simulink model "MLI"  (R2016a)
settings: Solver=VariableStepAuto  StartTime=0.0  StopTime=10  RelTol=1e-3
libraries: powerlib x26, powerlib_meascontrol x5, simulink x1
settings Model: Creator=Alin anto  LastModifiedBy=Alin anto

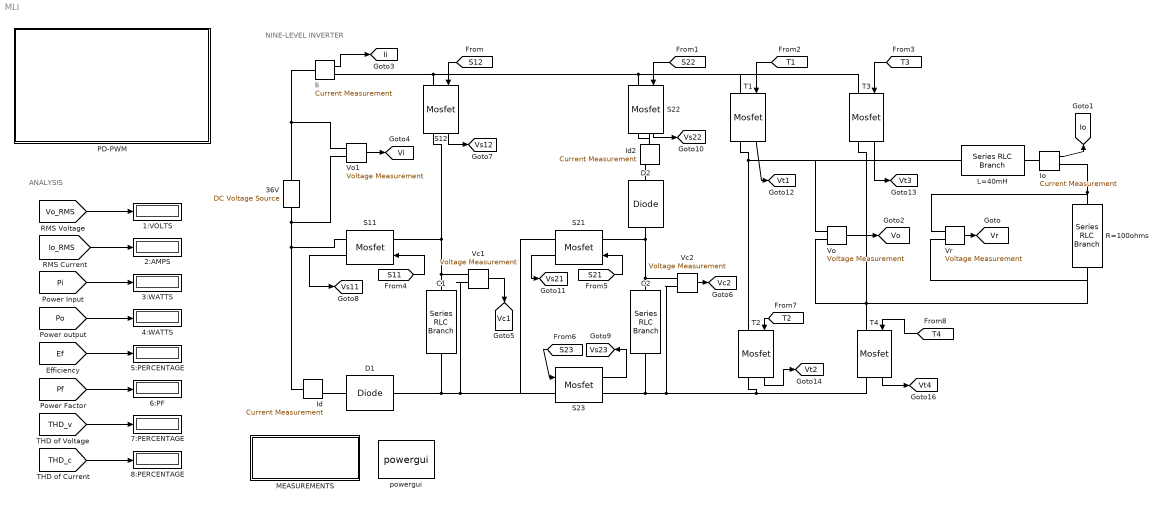
== system MLI ==
  note: ANALYSIS
  note: NINE-LEVEL INVERTER
  1:VOLTS : Display
  2:AMPS : Display
  36V : powerlib/Electrical Sources/DC Voltage Source  Amplitude=36  Measurements=None
  3:WATTS : Display
  4:WATTS : Display
  5:PERCENTAGE : Display
  6:PF : Display
  7:PERCENTAGE : Display
  8:PERCENTAGE : Display
  C1 : powerlib/Elements/Series RLC Branch  LConnTagsString=__new0  RConnTagsString=__new0  BranchType=C  Resistance=1  Inductance=1e-3  SetiL0=off  InitialCurrent=0  Capacitance=0.0024  Setx0=off  InitialVoltage=0  Measurements=None
  C2 : powerlib/Elements/Series RLC Branch  LConnTagsString=__new0  RConnTagsString=__new0  BranchType=C  Resistance=1  Inductance=1e-3  SetiL0=off  InitialCurrent=0  Capacitance=0.0036  Setx0=off  InitialVoltage=0  Measurements=None
  D1 : powerlib/Power Electronics/Diode  Ron=0.001  Lon=0  Vf=0.8  IC=0  UseSnubber=off  Rs=500  Cs=250e-9  Measurements=off
  D2 : powerlib/Power Electronics/Diode  Ron=0.001  Lon=0  Vf=0.8  IC=0  UseSnubber=off  Rs=500  Cs=250e-9  Measurements=off
  Id : powerlib/Measurements/Current Measurement  PhasorSimulation=off  OutputType=Complex  PSBequivalent=0
  Id2 : powerlib/Measurements/Current Measurement  PhasorSimulation=off  OutputType=Complex  PSBequivalent=0
  Ii : powerlib/Measurements/Current Measurement  PhasorSimulation=off  OutputType=Complex  PSBequivalent=0
  Io : powerlib/Measurements/Current Measurement  PhasorSimulation=off  OutputType=Complex  PSBequivalent=0
  L=40mH : powerlib/Elements/Series RLC Branch  LConnTagsString=__new0  RConnTagsString=__new0  BranchType=L  Resistance=1  Inductance=0.040  SetiL0=off  InitialCurrent=0  Capacitance=1e-6  Setx0=off  InitialVoltage=0  Measurements=None
  MEASUREMENTS : Subsystem
  PD-PWM : Subsystem
  R=100ohms : powerlib/Elements/Series RLC Branch  LConnTagsString=__new0  RConnTagsString=__new0  BranchType=R  Resistance=100  Inductance=1e-3  SetiL0=off  InitialCurrent=0  Capacitance=1e-6  Setx0=off  InitialVoltage=0  Measurements=None
  S{11..12,21..23} (5 alike) : powerlib/Power Electronics/Mosfet  Ron=0.1  Lon=0  Rd=0.01  Vfd=0.7  IC=0  Rs=1e5  Cs=inf  Measurements=on
  T{1..4} (4 alike) : powerlib/Power Electronics/Mosfet  Ron=0.1  Lon=0  Rd=0.01  Vfd=0.7  IC=0  Rs=1e5  Cs=inf  Measurements=on
  Vc1 : powerlib/Measurements/Voltage Measurement  PhasorSimulation=off  OutputType=Complex  PSBequivalent=0
  Vc2 : powerlib/Measurements/Voltage Measurement  PhasorSimulation=off  OutputType=Complex  PSBequivalent=0
  Vo : powerlib/Measurements/Voltage Measurement  PhasorSimulation=off  OutputType=Complex  PSBequivalent=0
  Vo1 : powerlib/Measurements/Voltage Measurement  PhasorSimulation=off  OutputType=Complex  PSBequivalent=0
  Vr : powerlib/Measurements/Voltage Measurement  PhasorSimulation=off  OutputType=Complex  PSBequivalent=0
  powergui : powerlib/powergui  Priority=1  SimulationMode=Discrete  SolverType=Tustin/Backward Euler (TBE)  SampleTime=1e-6  frequency=60  SPID=off  DisableSnubberDevices=off  DisableRonSwitches=off  DisableVfSwitches=off  SwTol=0  DisplayEquations=off  Interpol=off  ExternalGateDelay=off  methode=off  Ts=10  FunctionMessages=off  echomessages=off  HookPort=off  EnableUseOfTLC=off  x0status=blocks  frequencyindice=0  Pbase=100e6  ErrMax=1e-4  Iterations=50  UnitsV=kV  UnitsW=MW  buscounter=0  RestoreLinks=warning  ResistiveCurrentMeasurement=off  Frange=[0:2:500]  Ylog=off  Xlog=on  ShowGrid=off  save=off  variable=ZData  structure=FFT  ZoomFFT=on  StartTime=0.3  cycles=5  DisplayStyle=1  fundamental=50  FreqAxis=off  MaxFrequency=10000  frequencyindicesteady=1  RmsSteady=1  display=off
  tag scope: Ii=global, Io=global, Vc1=global, Vc2=global, Vi=global, Vo=global, Vr=global, Vs11=global, Vs12=global, Vs21=global, Vs22=global, Vs23=global, Vt1=global, Vt2=global, Vt3=global, Vt4=global
  wires:
  [T2] -> T2/1
  [S22] -> S22/1
  [S21] -> S21/1
  [T4] -> T4/1
  [S12] -> S12/1
  [S23] -> S23/1
  [T1] -> T1/1
  [S11] -> S11/1
  [T3] -> T3/1
  Io/1 -> [Io]
  Vo/1 -> [Vo]
  Vr/1 -> [Vr]
  Ii/1 -> [Ii]
  Vo1/1 -> [Vi]
  [Pi] -> 3:WATTS/1
  [THD_v] -> 7:PERCENTAGE/1
  [Pf] -> 6:PF/1
  [Ef] -> 5:PERCENTAGE/1
  [Po] -> 4:WATTS/1
  [THD_c] -> 8:PERCENTAGE/1
  [Io_RMS] -> 2:AMPS/1
  [Vo_RMS] -> 1:VOLTS/1
  Vc2/1 -> [Vc2]
  Vc1/1 -> [Vc1]
  S12/1 -> [Vs12]
  S11/1 -> [Vs11]
  S23/1 -> [Vs23]
  S22/1 -> [Vs22]
  S21/1 -> [Vs21]
  T4/1 -> [Vt4]
  T2/1 -> [Vt2]
  T1/1 -> [Vt1]
  T3/1 -> [Vt3]
  connections:
  S12/LConn1 -- Ii/RConn1 -- T3/LConn1 -- T1/LConn1 -- S22/LConn1
  L=40mH/RConn1 -- Io/LConn1
  T1/RConn1 -- Vo/LConn1 -- L=40mH/LConn1 -- T2/LConn1
  S23/RConn1 -- C2/RConn1 -- Vc2/LConn2 -- T2/RConn1 -- T4/RConn1
  36V/LConn1 -- Vo1/LConn2 -- Id/LConn1 -- S11/RConn1
  D1/LConn1 -- S21/RConn1 -- S23/LConn1 -- Vc1/LConn2 -- C1/RConn1
  C1/LConn1 -- S11/LConn1 -- S12/RConn1 -- Vc1/LConn1
  C2/LConn1 -- Vc2/LConn1 -- D2/RConn1 -- S21/LConn1
  Io/RConn1 -- Vr/LConn1 -- R=100ohms/LConn1
  T3/RConn1 -- R=100ohms/RConn1 -- Vr/LConn2 -- Vo/LConn2 -- T4/LConn1
  36V/RConn1 -- Vo1/LConn1 -- Ii/LConn1
  Id/RConn1 -- D1/RConn1
  Id2/RConn1 -- D2/LConn1
  Id2/LConn1 -- S22/RConn1

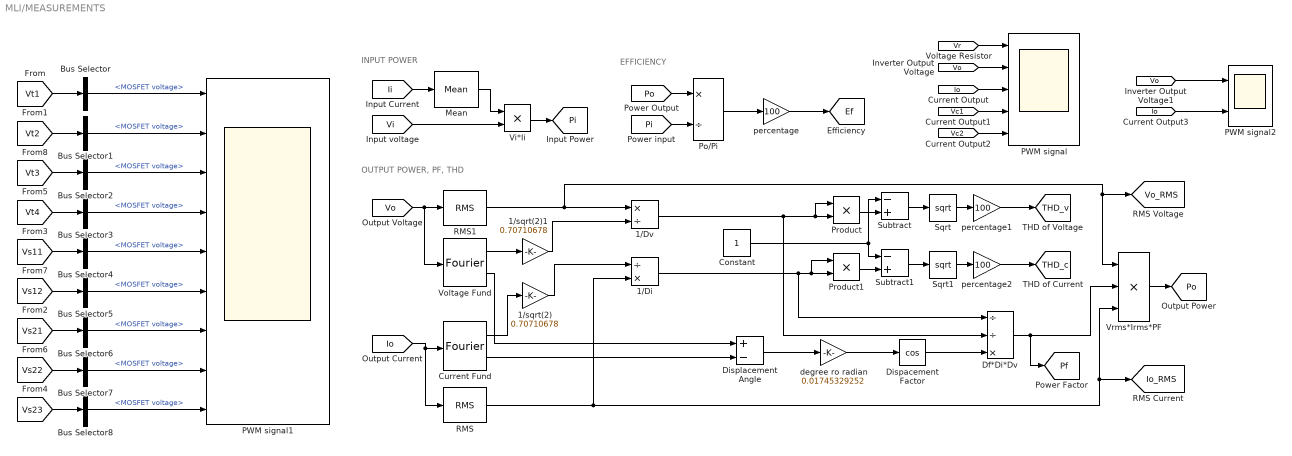
== system MLI/MEASUREMENTS ==
  note: OUTPUT POWER, PF, THD
  note: EFFICIENCY
  note: INPUT POWER
  1/Di : Product  Inputs=/*
  1/Dv : Product  Inputs=*/
  1/sqrt(2) : Gain  Gain=0.70710678
  1/sqrt(2)1 : Gain  Gain=0.70710678
  Bus Selector{,1..8} (9 alike) : BusSelector  OutputSignals=MOSFET voltage
  Constant : Constant
  Current Fund : powerlib_meascontrol/Measurements/Fourier  Freq=50  n=1  InInit=[120, 0]  Ts=0
  Df*Di*Dv : Product  Inputs=//*
  Dispacement Factor : Trigonometry  Operator=cos
  Displacement Angle : Sum  Inputs=+-
  Mean : powerlib_meascontrol/Measurements/Mean  Freq=50  Vinit=1  Ts=0
  PWM signal : Scope  NumInputPorts=5
  PWM signal1 : Scope  NumInputPorts=9
  PWM signal2 : Scope  NumInputPorts=2
  Po/Pi : Product  Inputs=*/
  Product : Product
  Product1 : Product
  RMS : powerlib_meascontrol/Measurements/RMS  TrueRMS=on  Freq=50  RMSInit=120  Ts=0
  RMS1 : powerlib_meascontrol/Measurements/RMS  TrueRMS=on  Freq=50  RMSInit=120  Ts=0
  Sqrt : Sqrt  SaturateOnIntegerOverflow=on
  Sqrt1 : Sqrt  SaturateOnIntegerOverflow=on
  Subtract : Sum  Inputs=-+
  Subtract1 : Sum  Inputs=-+
  Vi*Ii : Product
  Voltage Fund : powerlib_meascontrol/Measurements/Fourier  Freq=50  n=1  InInit=[120, 0]  Ts=0
  Vrms*Irms*PF : Product  Inputs=3
  degree ro radian : Gain  Gain=0.01745329252
  percentage : Gain  Gain=100
  percentage1 : Gain  Gain=100
  percentage2 : Gain  Gain=100
  tag scope: Ef=global, Io_RMS=global, Pf=global, Pi=global, Po=global, THD_c=global, THD_v=global, Vo_RMS=global
  wires:
  [Ii] -> Mean/1
  Mean/1 -> Vi*Ii/1
  [Vi] -> Vi*Ii/2
  Vi*Ii/1 -> [Pi]
  [Io] -> RMS/1, Current Fund/1
  Current Fund/1 -> 1/sqrt(2)/1
  RMS/1 -> [Io_RMS], Vrms*Irms*PF/3, 1/Di/2
  [Vo] -> Voltage Fund/1, RMS1/1
  Voltage Fund/1 -> 1/sqrt(2)1/1
  RMS1/1 -> [Vo_RMS], Vrms*Irms*PF/1, 1/Dv/1
  Voltage Fund/2 -> Displacement Angle/1
  Current Fund/2 -> Displacement Angle/2
  Displacement Angle/1 -> degree ro radian/1
  degree ro radian/1 -> Dispacement Factor/1
  1/Dv/1 -> Product/2, Product/1, Df*Di*Dv/2
  1/Di/1 -> Product1/1, Product1/2, Df*Di*Dv/1
  Df*Di*Dv/1 -> [Pf], Vrms*Irms*PF/2
  1/sqrt(2)1/1 -> 1/Dv/2
  Vrms*Irms*PF/1 -> [Po]
  Product/1 -> Subtract/2
  Constant/1 -> Subtract/1, Subtract1/1
  Subtract/1 -> Sqrt/1
  Subtract1/1 -> Sqrt1/1
  [Po] -> Po/Pi/1
  [Pi] -> Po/Pi/2
  Po/Pi/1 -> percentage/1
  percentage/1 -> [Ef]
  Sqrt/1 -> percentage1/1
  percentage1/1 -> [THD_v]
  Sqrt1/1 -> percentage2/1
  percentage2/1 -> [THD_c]
  [Vr] -> PWM signal/1
  [Vo] -> PWM signal/2
  [Io] -> PWM signal/3
  1/sqrt(2)/1 -> 1/Di/1
  Product1/1 -> Subtract1/2
  Dispacement Factor/1 -> Df*Di*Dv/3
  [Vc1] -> PWM signal/4
  [Vc2] -> PWM signal/5
  [Vt1] -> Bus Selector/1
  [Vt2] -> Bus Selector1/1
  [Vt3] -> Bus Selector2/1
  [Vt4] -> Bus Selector3/1
  [Vs11] -> Bus Selector4/1
  [Vs12] -> Bus Selector5/1
  [Vs21] -> Bus Selector6/1
  [Vs22] -> Bus Selector7/1
  [Vs23] -> Bus Selector8/1
  Bus Selector/1 -> PWM signal1/1  "<MOSFET voltage>"
  Bus Selector1/1 -> PWM signal1/2  "<MOSFET voltage>"
  Bus Selector2/1 -> PWM signal1/3  "<MOSFET voltage>"
  Bus Selector3/1 -> PWM signal1/4  "<MOSFET voltage>"
  Bus Selector4/1 -> PWM signal1/5  "<MOSFET voltage>"
  Bus Selector5/1 -> PWM signal1/6  "<MOSFET voltage>"
  Bus Selector6/1 -> PWM signal1/7  "<MOSFET voltage>"
  Bus Selector7/1 -> PWM signal1/8  "<MOSFET voltage>"
  Bus Selector8/1 -> PWM signal1/9  "<MOSFET voltage>"
  [Vo] -> PWM signal2/1
  [Io] -> PWM signal2/2

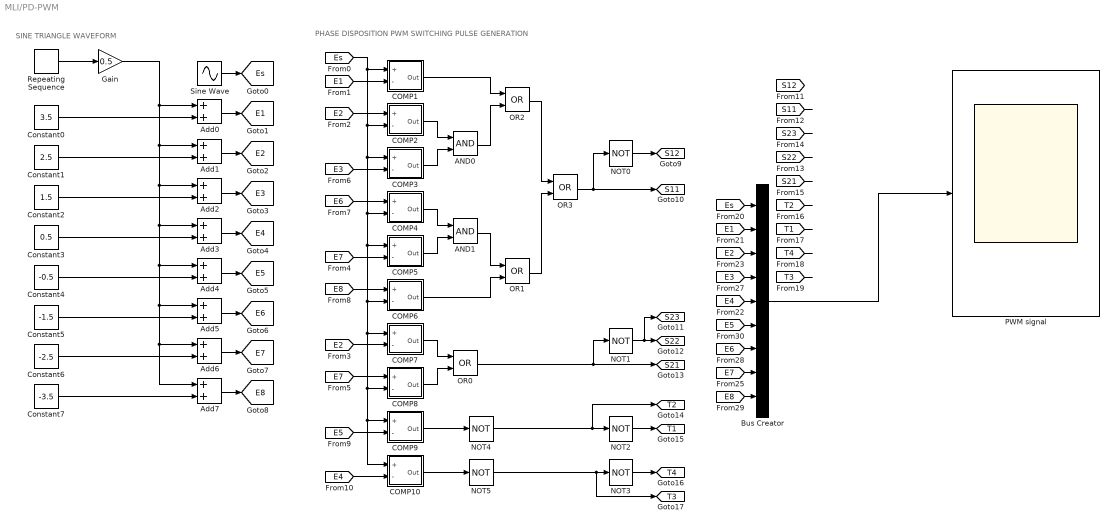
== system MLI/PD-PWM ==
  note: PHASE DISPOSITION PWM SWITCHING PULSE GENERATION
  note: SINE TRIANGLE WAVEFORM
  AND0 : Logic  AllPortsSameDT=off  OutDataTypeStr=boolean
  AND1 : Logic  AllPortsSameDT=off  OutDataTypeStr=boolean
  Add{0..7} (8 alike) : Sum
  Bus Creator : BusCreator  Inputs=9
  COMP1 : Subsystem
  COMP10 : Subsystem
  COMP2 : Subsystem
  COMP3 : Subsystem
  COMP4 : Subsystem
  COMP5 : Subsystem
  COMP6 : Subsystem
  COMP7 : Subsystem
  COMP8 : Subsystem
  COMP9 : Subsystem
  Constant0 : Constant  Value=3.5
  Constant1 : Constant  Value=2.5
  Constant2 : Constant  Value=1.5
  Constant3 : Constant  Value=0.5
  Constant4 : Constant  Value=-0.5
  Constant5 : Constant  Value=-1.5
  Constant6 : Constant  Value=-2.5
  Constant7 : Constant  Value=-3.5
  Gain : Gain  Gain=0.5
  NOT{0..5} (6 alike) : Logic  Operator=NOT  AllPortsSameDT=off  OutDataTypeStr=boolean
  OR{0..3} (4 alike) : Logic  Operator=OR  AllPortsSameDT=off  OutDataTypeStr=boolean
  PWM signal : Scope
  Repeating Sequence : simulink/Sources/Repeating Sequence  rep_seq_t=[0 5e-5 15e-5 20e-5]  rep_seq_y=[0 1 -1 0]
  Sine Wave : Sin  Amplitude=4  Frequency=2*pi*50  SampleTime=0
  tag scope: E1=global, E2=global, E3=global, E4=global, E5=global, E6=global, E7=global, E8=global, Es=global, S11=global, S12=global, S21=global, S22=global, S23=global, T1=global, T2=global, T3=global, T4=global
  wires:
  COMP1/1(Out) -> OR2/1
  OR0/1 -> [S21], NOT1/1
  OR3/1 -> [S11], NOT0/1
  OR2/1 -> OR3/1
  OR1/1 -> OR3/2
  NOT1/1 -> [S22], [S23]
  NOT0/1 -> [S12]
  COMP4/1(Out) -> AND1/1
  COMP7/1(Out) -> OR0/1
  COMP2/1(Out) -> AND0/1
  COMP6/1(Out) -> OR1/2
  AND0/1 -> OR2/2
  COMP3/1(Out) -> AND0/2
  COMP5/1(Out) -> AND1/2
  AND1/1 -> OR1/1
  COMP8/1(Out) -> OR0/2
  [Es] -> COMP4/2(-), COMP6/2(-), COMP7/1(+), COMP8/2(-), COMP9/1(+), COMP10/1(+), COMP5/1(+), COMP3/1(+), COMP2/2(-), COMP1/1(+)
  [E1] -> COMP1/2(-)
  [E2] -> COMP2/1(+)
  [E3] -> COMP3/2(-)
  [E6] -> COMP4/1(+)
  [E7] -> COMP5/2(-)
  [E8] -> COMP6/1(+)
  [E5] -> COMP9/2(-)
  [E4] -> COMP10/2(-)
  COMP9/1(Out) -> NOT4/1
  NOT4/1 -> [T2], NOT2/1
  NOT2/1 -> [T1]
  COMP10/1(Out) -> NOT5/1
  NOT5/1 -> [T3], NOT3/1
  NOT3/1 -> [T4]
  Constant2/1 -> Add2/2
  Constant3/1 -> Add3/2
  Constant0/1 -> Add0/2
  Constant1/1 -> Add1/2
  Repeating Sequence/1 -> Gain/1
  Gain/1 -> Add7/1, Add6/1, Add5/1, Add4/1, Add3/1, Add2/1, Add1/1, Add0/1
  Constant4/1 -> Add4/2
  Constant6/1 -> Add6/2
  Constant7/1 -> Add7/2
  Constant5/1 -> Add5/2
  Sine Wave/1 -> [Es]
  Add0/1 -> [E1]
  Add1/1 -> [E2]
  Add2/1 -> [E3]
  Add7/1 -> [E8]
  Add6/1 -> [E7]
  Add5/1 -> [E6]
  Add4/1 -> [E5]
  Add3/1 -> [E4]
  [E2] -> COMP7/2(-)
  [E7] -> COMP8/1(+)
  [S23] -> ?
  [S22] -> ?
  [S21] -> ?
  [T2] -> ?
  [T1] -> ?
  [T4] -> ?
  [T3] -> ?
  [S11] -> ?
  [Es] -> Bus Creator/1
  [E1] -> Bus Creator/2
  [E2] -> Bus Creator/3
  [E3] -> Bus Creator/4
  [E4] -> Bus Creator/5
  [E5] -> Bus Creator/6
  [E6] -> Bus Creator/7
  [E7] -> Bus Creator/8
  [E8] -> Bus Creator/9
  Bus Creator/1 -> PWM signal/1

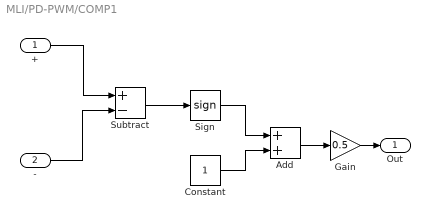
== system MLI/PD-PWM/COMP1 ==
  + : Inport
  - : Inport  Port=2
  Add : Sum
  Constant : Constant
  Gain : Gain  Gain=0.5
  Sign : Signum
  Subtract : Sum  Inputs=+-
  Out : Outport
  wires:
  Add/1 -> Gain/1
  -/1 -> Subtract/2
  Gain/1 -> Out/1
  +/1 -> Subtract/1
  Constant/1 -> Add/2
  Sign/1 -> Add/1
  Subtract/1 -> Sign/1

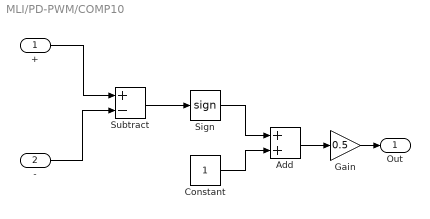
== system MLI/PD-PWM/COMP10 ==
  + : Inport
  - : Inport  Port=2
  Add : Sum
  Constant : Constant
  Gain : Gain  Gain=0.5
  Sign : Signum
  Subtract : Sum  Inputs=+-
  Out : Outport
  wires:
  Add/1 -> Gain/1
  -/1 -> Subtract/2
  Gain/1 -> Out/1
  +/1 -> Subtract/1
  Constant/1 -> Add/2
  Sign/1 -> Add/1
  Subtract/1 -> Sign/1

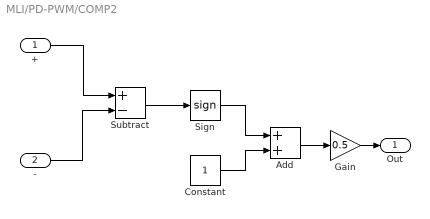
== system MLI/PD-PWM/COMP2 ==
  + : Inport
  - : Inport  Port=2
  Add : Sum
  Constant : Constant
  Gain : Gain  Gain=0.5
  Sign : Signum
  Subtract : Sum  Inputs=+-
  Out : Outport
  wires:
  Add/1 -> Gain/1
  -/1 -> Subtract/2
  Gain/1 -> Out/1
  +/1 -> Subtract/1
  Constant/1 -> Add/2
  Sign/1 -> Add/1
  Subtract/1 -> Sign/1

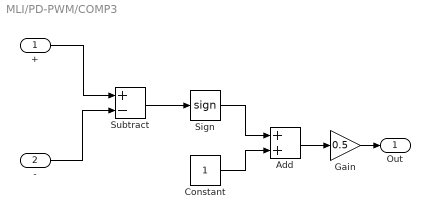
== system MLI/PD-PWM/COMP3 ==
  + : Inport
  - : Inport  Port=2
  Add : Sum
  Constant : Constant
  Gain : Gain  Gain=0.5
  Sign : Signum
  Subtract : Sum  Inputs=+-
  Out : Outport
  wires:
  Add/1 -> Gain/1
  -/1 -> Subtract/2
  Gain/1 -> Out/1
  +/1 -> Subtract/1
  Constant/1 -> Add/2
  Sign/1 -> Add/1
  Subtract/1 -> Sign/1

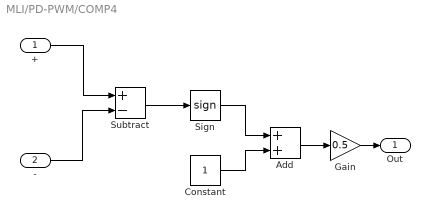
== system MLI/PD-PWM/COMP4 ==
  + : Inport
  - : Inport  Port=2
  Add : Sum
  Constant : Constant
  Gain : Gain  Gain=0.5
  Sign : Signum
  Subtract : Sum  Inputs=+-
  Out : Outport
  wires:
  Add/1 -> Gain/1
  -/1 -> Subtract/2
  Gain/1 -> Out/1
  +/1 -> Subtract/1
  Constant/1 -> Add/2
  Sign/1 -> Add/1
  Subtract/1 -> Sign/1

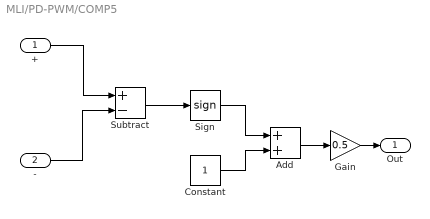
== system MLI/PD-PWM/COMP5 ==
  + : Inport
  - : Inport  Port=2
  Add : Sum
  Constant : Constant
  Gain : Gain  Gain=0.5
  Sign : Signum
  Subtract : Sum  Inputs=+-
  Out : Outport
  wires:
  Add/1 -> Gain/1
  -/1 -> Subtract/2
  Gain/1 -> Out/1
  +/1 -> Subtract/1
  Constant/1 -> Add/2
  Sign/1 -> Add/1
  Subtract/1 -> Sign/1

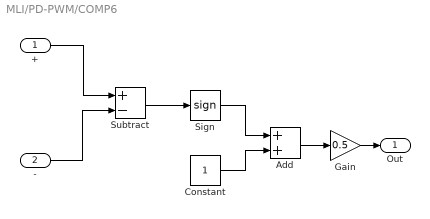
== system MLI/PD-PWM/COMP6 ==
  + : Inport
  - : Inport  Port=2
  Add : Sum
  Constant : Constant
  Gain : Gain  Gain=0.5
  Sign : Signum
  Subtract : Sum  Inputs=+-
  Out : Outport
  wires:
  Add/1 -> Gain/1
  -/1 -> Subtract/2
  Gain/1 -> Out/1
  +/1 -> Subtract/1
  Constant/1 -> Add/2
  Sign/1 -> Add/1
  Subtract/1 -> Sign/1

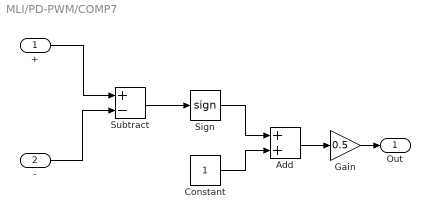
== system MLI/PD-PWM/COMP7 ==
  + : Inport
  - : Inport  Port=2
  Add : Sum
  Constant : Constant
  Gain : Gain  Gain=0.5
  Sign : Signum
  Subtract : Sum  Inputs=+-
  Out : Outport
  wires:
  Add/1 -> Gain/1
  -/1 -> Subtract/2
  Gain/1 -> Out/1
  +/1 -> Subtract/1
  Constant/1 -> Add/2
  Sign/1 -> Add/1
  Subtract/1 -> Sign/1

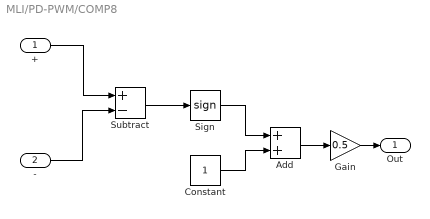
== system MLI/PD-PWM/COMP8 ==
  + : Inport
  - : Inport  Port=2
  Add : Sum
  Constant : Constant
  Gain : Gain  Gain=0.5
  Sign : Signum
  Subtract : Sum  Inputs=+-
  Out : Outport
  wires:
  Add/1 -> Gain/1
  -/1 -> Subtract/2
  Gain/1 -> Out/1
  +/1 -> Subtract/1
  Constant/1 -> Add/2
  Sign/1 -> Add/1
  Subtract/1 -> Sign/1

== system MLI/PD-PWM/COMP9 ==
  + : Inport
  - : Inport  Port=2
  Add : Sum
  Constant : Constant
  Gain : Gain  Gain=0.5
  Sign : Signum
  Subtract : Sum  Inputs=+-
  Out : Outport
  wires:
  Add/1 -> Gain/1
  -/1 -> Subtract/2
  Gain/1 -> Out/1
  +/1 -> Subtract/1
  Constant/1 -> Add/2
  Sign/1 -> Add/1
  Subtract/1 -> Sign/1
